simulink model "PMSM_2017b_1013"  (R2017b)
settings: Solver=FixedStepDiscrete  StartTime=0.0  StopTime=0.4  FixedStep=Ts  RelTol=1e-4  EnableMultiTasking=on
values from neighbouring files (symbols this model uses):
  AgSelector = 0    [initialization_1013.m]
  Ba = (Beta*J- Fl)/(1.5*P*flux)    [initialization_1013.m]
  Fl = 0.007*3/(100*pi)    (= 6.68450760986e-05)    [initialization_1013.m]
  flux = Kt/(1.5*P*sqrt(2))    [initialization_1013.m]
  fpwm = 1e4    (= 10000)    [initialization_1013.m]
  Imax = 6*sqrt(2)    [initialization_1013.m]
  J = 9.96e-5    (= 9.96e-05)    [initialization_1013.m]
  K1 = wn^2    (= 1000000)    [initialization_1013.m]
  K2 = 2*fei/wn    (= 0.003)    [initialization_1013.m]
  K_resolver = 1    [initialization_1013.m]
  Ki_Cctrl_d = Rs/(4*Tpwm)    (= 22125)    [initialization_1013.m]
  Ki_Cctrl_q = Rs/(4*Tpwm)    (= 22125)    [initialization_1013.m]
  Ki_Spdctrl = Beta*Kp_Spdctrl    [initialization_1013.m]
  Ki_Spdctrl_2 = 0.12*(pi*J)/(6000*P*flux*Tpwm^2)    [initialization_1013.m]
  Kp_Cctrl_d = Ld/(4*Tpwm)    (= 231.25)    [initialization_1013.m]
  Kp_Cctrl_q = Lq/(4*Tpwm)    (= 231.25)    [initialization_1013.m]
  Kp_Spdctrl = (Beta*J)/(1.5*P*flux)    [initialization_1013.m]
  Kp_Spdctrl_2 = 1*(pi*J)/(300*P*flux*Tpwm)    [initialization_1013.m]
  Kt = 1.32    [initialization_1013.m]
  Ld = Ls    (= 0.0925)    [initialization_1013.m]
  Lq = Ls    (= 0.0925)    [initialization_1013.m]
  Ls = 0.185/2    (= 0.0925)    [initialization_1013.m]
  P = 2    [initialization_1013.m]
  Rs = 17.7/2    (= 8.85)    [initialization_1013.m]
  SimMode = 1    [initialization_1013.m]
  TestCurrentController = 0    [initialization_1013.m]
  Tf = 0.08    [initialization_1013.m]
  Tpwm = 1e-4    (= 0.0001)    [initialization_1013.m]
  TqNorm = 0.6*9550/2500    (= 2.292)    [initialization_1013.m]
  Ts = 1e-6    (= 1e-06)    [initialization_1013.m]
  Udc = 230*sqrt(2)    [initialization_1013.m]
undefined symbols (not defined in the file or in its folder): A, B, DiscIntNeverNeededParam, f_LPF, f_LPF2, Init, K_SMO, Ki, Ki_PLL_SMO, Kp, Kp_PLL_SMO, LowerLimit, rate, UpperLimit
libraries: simulink x11, powerlib x7
(part 2 of 2)

== system PMSM_2017b_1013/SW/AgWeCalculation/Ag_atan2 ==
  Sin : Inport
  cos : Inport  Port=2
  Discrete Derivative : simulink/Discrete/Discrete Derivative  gainval=1.0  ICPrevScaledInput=0.0  OutMin=[]  OutMax=[]  OutDataType=fixdt(1, 16)  OutScaling=2^-10  DoSatur=off
  Sin1 : Trigonometry  Operator=atan2
  Ag : Outport
  we : Outport  Port=2
  wires:
  Sin/1 -> Sin1/1
  Sin1/1 -> Discrete Derivative/1, Ag/1
  Discrete Derivative/1 -> we/1
  cos/1 -> Sin1/2

== system PMSM_2017b_1013/SW/AgWeCalculation/LPF1 ==
  u_in : Inport
  Add : Sum  Inputs=+-
  Add1 : Sum
  Constant : Constant  Value=Tpwm
  Constant1 : Constant  Value=3000/(2*pi)
  Gain3 : Gain  Gain=2*pi
  Product : Product
  Product1 : Product
  Scope_We{1..4} (4 alike) : Scope
  Unit Delay : UnitDelay  SampleTime=-1
  u_out : Outport
  wires:
  Add1/1 -> Unit Delay/1, Scope_We2/1, u_out/1
  Product/1 -> Product1/1
  Add/1 -> Scope_We3/1, Product1/2
  Product1/1 -> Scope_We1/1, Add1/1
  Gain3/1 -> Product/2
  Constant/1 -> Product/1
  Constant1/1 -> Gain3/1
  u_in/1 -> Scope_We4/1, Add/1
  Unit Delay/1 -> Add/2, Add1/2

== system PMSM_2017b_1013/SW/AgWeCalculation/UseRslvrAg ==
  Rslvr_Sin : Inport
  Rslvr_Cos : Inport  Port=2
  Ag_PIcontroller : Subsystem
  Ag_Rslvr : Outport
  We__Rslvr : Outport  Port=2
  wires:
  Rslvr_Sin/1 -> Ag_PIcontroller/1(In1)
  Rslvr_Cos/1 -> Ag_PIcontroller/2(In2)
  Ag_PIcontroller/2(we) -> We__Rslvr/1
  Ag_PIcontroller/1(Ag) -> Ag_Rslvr/1

== system PMSM_2017b_1013/SW/AgWeCalculation/UseSimAg ==
  Agm : Inport
  wm : Inport  Port=2
  Agm2Ag : Gain  Gain=P
  Constant2 : Constant  Value=2*pi
  Mod : Math  Operator=mod  SaturateOnIntegerOverflow=on
  wm2we : Gain  Gain=P
  Ag_sim : Outport
  We_sim : Outport  Port=2
  wires:
  wm2we/1 -> We_sim/1  "we_sim"
  Agm/1 -> Agm2Ag/1
  wm/1 -> wm2we/1
  Agm2Ag/1 -> Mod/1  "Ag_sim"
  Constant2/1 -> Mod/2
  Mod/1 -> Ag_sim/1

== system PMSM_2017b_1013/SW/CurrentController/Anti_Clark ==
  UAlphaBeta : Inport
  Fcn : Fcn  Expr=-0.5*u(1)+sqrt(3)/2*u(2)
  Fcn1 : Fcn  Expr=-0.5*u(1)-sqrt(3)/2*u(2)
  Fcn2 : Fcn  Expr=u(1)
  Mux : Mux  Inputs=3
  Uabc : Outport
  wires:
  UAlphaBeta/1 -> Fcn1/1, Fcn2/1, Fcn/1
  Mux/1 -> Uabc/1
  Fcn2/1 -> Mux/1
  Fcn/1 -> Mux/2
  Fcn1/1 -> Mux/3

== system PMSM_2017b_1013/SW/CurrentController/Anti_Park ==
  Udq : Inport
  Ag : Inport  Port=2
  Constant3 : Constant  Value=1/10000
  ConstantAg : Constant
  Fcn : Fcn  Expr=u(1)*cos(u(3))-u(2)*sin(u(3))
  Fcn1 : Fcn  Expr=u(1)*sin(u(3))+u(2)*cos(u(3))
  Multiport Switch : MultiPortSwitch
  Mux : Mux  Inputs=2
  Mux1 : Mux  Inputs=2
  Mux2 : Mux  Inputs=3
  Sum : Sum  Inputs=|++
  Switch : Switch  Criteria=u2 > Threshold  Threshold=0.5
  SwitchAgForOpenLoop : Constant
  SwitchOpenLoop : Constant  Value=0
  Ud_Inject : Constant  Value=0
  Unit Delay : UnitDelay  SampleTime=-1
  Uq_Inject : Constant  Value=0
  UAlphaBeta : Outport
  wires:
  Udq/1 -> Mux1/1
  Switch/1 -> Fcn1/1, Fcn/1
  Uq_Inject/1 -> Mux2/2
  Mux2/1 -> Switch/1
  Mux1/1 -> Switch/3
  SwitchOpenLoop/1 -> Switch/2
  Ud_Inject/1 -> Mux2/1
  Constant3/1 -> Sum/1
  Unit Delay/1 -> Sum/2
  Sum/1 -> Unit Delay/1, Multiport Switch/3
  Ag/1 -> Multiport Switch/4, Mux1/2
  Fcn/1 -> Mux/1
  Fcn1/1 -> Mux/2
  Mux/1 -> UAlphaBeta/1
  Multiport Switch/1 -> Mux2/3
  SwitchAgForOpenLoop/1 -> Multiport Switch/1
  ConstantAg/1 -> Multiport Switch/2

== system PMSM_2017b_1013/SW/CurrentController/Clamping_PI ==
  Idq_error : Inport
  Udc : Inport  Port=2
  Clamping_PI_d : Subsystem
  Clamping_PI_q : Subsystem
  Constant : Constant  Value=Kp_Cctrl_d
  Constant1 : Constant  Value=Ki_Cctrl_d
  Constant2 : Constant  Value=Kp_Cctrl_q
  Constant3 : Constant  Value=Ki_Cctrl_q
  Demux : Demux  Outputs=2
  Mux : Mux  Inputs=2
  Udq_pi : Outport  InitialOutput=0
  wires:
  Idq_error/1 -> Demux/1
  Demux/1 -> Clamping_PI_d/1(Error)
  Clamping_PI_d/1(Out) -> Mux/1
  Mux/1 -> Udq_pi/1
  Udc/1 -> Clamping_PI_q/2(Udc), Clamping_PI_d/2(Udc)
  Constant/1 -> Clamping_PI_d/3(Kp)
  Constant1/1 -> Clamping_PI_d/4(Ki)
  Clamping_PI_q/1(Out) -> Mux/2
  Constant3/1 -> Clamping_PI_q/4(Ki)
  Constant2/1 -> Clamping_PI_q/3(Kp)
  Demux/2 -> Clamping_PI_q/1(Error)

== system PMSM_2017b_1013/SW/CurrentController/Clark ==
  Iabc : Inport
  Mux1 : Mux  Inputs=2
  alpha : Fcn  Expr=(u(1)-0.5*(u(2)+u(3)))*2/3
  beta : Fcn  Expr=sqrt(3)/2*(u(2)-u(3))*2/3
  I_AlphaBeta : Outport
  wires:
  Iabc/1 -> alpha/1, beta/1
  alpha/1 -> Mux1/1
  beta/1 -> Mux1/2
  Mux1/1 -> I_AlphaBeta/1

== system PMSM_2017b_1013/SW/CurrentController/Decoup ==
  IdqAct : Inport
  we : Inport  Port=2
  Fcn : Fcn  Expr=(u(1)*u(3)*Ld)+(u(3)*flux)
  Fcn1 : Fcn  Expr=-u(2)*u(3)*Lq
  Mux2 : Mux  Inputs=2
  Mux3 : Mux  Inputs=2
  Udq_decp : Outport
  wires:
  we/1 -> Mux2/2
  IdqAct/1 -> Mux2/1
  Fcn1/1 -> Mux3/1
  Fcn/1 -> Mux3/2
  Mux3/1 -> Udq_decp/1
  Mux2/1 -> Fcn1/1, Fcn/1

== system PMSM_2017b_1013/SW/CurrentController/Friction ==
  note: 参考： 摩擦力模型综述 - 豆丁网 (docin.com)
      | 库伦+粘滞摩擦模型： T = Tf * sgn(wm) + Fl*wm
      |
      | 实际转速在0附近会有波动，因此设定一个2rpm的范围，最大静摩擦扭矩与转速成近似线性。
      | 否则实际控制中，0转速会有dq电流在波动。
      |
      | 还有一种解决方案，通过测功机拖动被测电机，测试不同转速下的 摩擦扭矩。最终形成插值表。
      | (该方法对测功机低速控制要求较高)
  we : Inport
  Abs : Abs
  Add : Sum
  Constant : Constant  Value=0
  Divide : Product  Inputs=*/
  Mux1 : Mux  Inputs=2
  Nm->Iq : Gain  Gain=sqrt(2)/Kt
  Product : Product
  Product1 : Product
  Relational Operator : RelationalOperator  OutDataTypeStr=boolean  RndMeth=Simplest
  Rpm2wm : Gain  Gain=pi/30
  RpmThreshold : Constant  Value=2
  Scope1 : Scope
  Scope2 : Scope
  Sign : Signum
  Static : Constant  Value=Tf
  Switch1 : Switch  Criteria=u2 > Threshold  Threshold=0.5
  viscous : Gain  Gain=Fl
  we2wm : Gain  Gain=1/P
  Idq_Friction : Outport
  wires:
  we/1 -> we2wm/1
  viscous/1 -> Add/1
  Mux1/1 -> Idq_Friction/1
  Nm->Iq/1 -> Mux1/2
  Constant/1 -> Mux1/1
  we2wm/1 -> Product1/2, Abs/1, Sign/1, viscous/1, Scope1/1
  Abs/1 -> Relational Operator/1
  Relational Operator/1 -> Switch1/2
  Product/1 -> Add/2
  Add/1 -> Switch1/1
  Switch1/1 -> Scope2/1, Nm->Iq/1
  Sign/1 -> Product/2
  Product1/1 -> Switch1/3
  RpmThreshold/1 -> Divide/2, Rpm2wm/1
  Rpm2wm/1 -> Relational Operator/2
  Static/1 -> Divide/1, Product/1
  Divide/1 -> Product1/1

== system PMSM_2017b_1013/SW/CurrentController/Park ==
  I_AlphaBeta : Inport
  Ag : Inport  Port=2
  Mux : Mux  Inputs=2
  Mux1 : Mux  Inputs=2
  d : Fcn  Expr=u(1)*cos(u(3))+u(2)*sin(u(3))
  q : Fcn  Expr=-u(1)*sin(u(3))+u(2)*cos(u(3))
  IdqAct : Outport
  wires:
  I_AlphaBeta/1 -> Mux/1
  Mux/1 -> q/1, d/1
  Ag/1 -> Mux/2
  d/1 -> Mux1/1
  q/1 -> Mux1/2
  Mux1/1 -> IdqAct/1

== system PMSM_2017b_1013/SW/CurrentController/TqEstimation ==
  IdqAct : Inport
  Demux : Demux  Outputs=2
  Iq2Nm : Gain  Gain=Kt/sqrt(2)
  Scope2 : Scope
  Terminator : Terminator
  TqAct : Outport
  wires:
  Iq2Nm/1 -> TqAct/1, Scope2/1
  IdqAct/1 -> Demux/1
  Demux/2 -> Iq2Nm/1
  Demux/1 -> Terminator/1

== system PMSM_2017b_1013/SW/SVPWM/Sector Caculate ==
  Ualpha : Inport
  Ubeta : Inport  Port=2
  B0 : Fcn  Expr=u[2]
  B1 : Fcn  Expr=u[1]*sqrt(3/4)-0.5*u[2]
  B2 : Fcn  Expr=-u[1]*sqrt(3/4)-u[2]*0.5
  Constant : Constant
  Constant1 : Constant  Value=0
  Mux : Mux  Inputs=2
  Mux1 : Mux  Inputs=3
  N : Fcn  Expr=4*u[3]+2*u[2]+u[1]
  Switch : Switch
  Switch1 : Switch
  Switch2 : Switch
  "N " : Outport
  wires:
  Switch2/1 -> Mux1/3
  Switch/1 -> Mux1/1
  Ualpha/1 -> Mux/1
  Ubeta/1 -> Mux/2
  Mux/1 -> B2/1, B1/1, B0/1
  B0/1 -> Switch/2
  B1/1 -> Switch1/2
  B2/1 -> Switch2/2
  Constant/1 -> Switch/1, Switch2/1, Switch1/1
  Constant1/1 -> Switch/3, Switch1/3, Switch2/3
  Switch1/1 -> Mux1/2
  Mux1/1 -> N/1
  N/1 -> "N "/1

== system PMSM_2017b_1013/SW/SVPWM/T1T1 Caculate ==
  note: T1
  note: T2
  N : Inport
  XYZ : Inport  Port=2
  Tpwm : Inport  Port=3
  Demux : Demux  Outputs=3
  Fcn : Fcn  Expr=u(3)-u(2)-u(1)
  Fcn1 : Fcn  Expr=u(1)*u(3)/(u(1)+u(2))
  Fcn2 : Fcn  Expr=u(2)*u(3)/(u(1)+u(2))
  Gain : Gain  Gain=-1
  Gain1 : Gain  Gain=-1
  Gain2 : Gain  Gain=-1
  Multiport Switch : MultiPortSwitch  Inputs=6  DiagnosticForDefault=Warning
  Multiport Switch1 : MultiPortSwitch  Inputs=6  DiagnosticForDefault=Warning
  Mux : Mux  Inputs=3
  Switch : Switch
  Switch1 : Switch  Criteria=u2 > Threshold
  T1 : Outport
  T2 : Outport  Port=2
  wires:
  Tpwm/1 -> Mux/3
  XYZ/1 -> Demux/1
  Switch1/1 -> T2/1
  Switch/1 -> T1/1
  Fcn2/1 -> Switch1/3
  Fcn1/1 -> Switch/3
  Fcn/1 -> Switch/2, Switch1/2
  Mux/1 -> Fcn1/1, Fcn/1, Fcn2/1
  Multiport Switch/1 -> Switch/1, Mux/1
  Multiport Switch1/1 -> Switch1/1, Mux/2
  N/1 -> Multiport Switch/1, Multiport Switch1/1
  Demux/2 -> Multiport Switch/3, Multiport Switch1/2, Gain1/1
  Demux/3 -> Multiport Switch1/5, Multiport Switch/2, Gain2/1
  Demux/1 -> Multiport Switch/6, Multiport Switch1/4, Gain/1
  Gain/1 -> Multiport Switch1/3, Multiport Switch/5
  Gain2/1 -> Multiport Switch/4, Multiport Switch1/7
  Gain1/1 -> Multiport Switch1/6, Multiport Switch/7

== system PMSM_2017b_1013/SW/SVPWM/Tcm Caculate ==
  N : Inport
  T1 : Inport  Port=2
  T2 : Inport  Port=3
  Tpwm : Inport  Port=4
  Fcn : Fcn  Expr=(u[3]-u[1]-u[2])/4
  Fcn1 : Fcn  Expr=(u[3]+u[1]-u[2])/4
  Fcn2 : Fcn  Expr=(u[3]+u[2]+u[1])/4
  Multiport Switch : MultiPortSwitch  Inputs=6  DiagnosticForDefault=Warning
  Multiport Switch1 : MultiPortSwitch  Inputs=6  DiagnosticForDefault=Warning
  Multiport Switch2 : MultiPortSwitch  Inputs=6  DiagnosticForDefault=Warning
  Mux : Mux  Inputs=3
  Mux1 : Mux  Inputs=3
  Tcm1 Tcm2 Tcm3 : Outport
  wires:
  Mux/1 -> Fcn2/1, Fcn/1, Fcn1/1
  Tpwm/1 -> Mux/3
  T2/1 -> Mux/2
  T1/1 -> Mux/1
  Multiport Switch2/1 -> Mux1/3
  Multiport Switch1/1 -> Mux1/2
  Multiport Switch/1 -> Mux1/1
  Mux1/1 -> Tcm1 Tcm2 Tcm3/1
  Fcn/1 -> Multiport Switch/3, Multiport Switch/4, Multiport Switch1/6, Multiport Switch2/5, Multiport Switch2/7, Multiport Switch1/2
  Fcn1/1 -> Multiport Switch1/5, Multiport Switch2/3, Multiport Switch2/6, Multiport Switch1/4, Multiport Switch/7, Multiport Switch/2
  Fcn2/1 -> Multiport Switch/5, Multiport Switch/6, Multiport Switch1/3, Multiport Switch1/7, Multiport Switch2/2, Multiport Switch2/4
  N/1 -> Multiport Switch2/1, Multiport Switch1/1, Multiport Switch/1

== system PMSM_2017b_1013/SW/SVPWM/XYZ Caculate ==
  Ualpha : Inport
  Ubeta : Inport  Port=2
  Tpwm : Inport  Port=3
  Udc : Inport  Port=4
  Add : Sum
  Add1 : Sum  Inputs=+-
  Gain : Gain  Gain=3/2
  Gain1 : Gain  Gain=sqrt(3)
  Gain2 : Gain  Gain=sqrt(3)/2
  Math Function : Math  Operator=reciprocal  SaturateOnIntegerOverflow=on
  Mux : Mux  Inputs=3
  Product{,1..3} (4 alike) : Product  RndMeth=Zero
  XYZ : Outport
  wires:
  Mux/1 -> XYZ/1
  Product1/1 -> Mux/1
  Product3/1 -> Mux/2
  Product2/1 -> Mux/3
  Ualpha/1 -> Gain/1
  Ubeta/1 -> Gain2/1, Gain1/1
  Udc/1 -> Math Function/1
  Math Function/1 -> Product/2
  Tpwm/1 -> Product/1
  Gain1/1 -> Product1/1
  Product/1 -> Product2/2, Product1/2, Product3/2
  Gain/1 -> Add1/2, Add/2
  Gain2/1 -> Add/1, Add1/1
  Add1/1 -> Product2/1
  Add/1 -> Product3/1

== system PMSM_2017b_1013/SW/SpdController/Clamping_PI ==
  Spd_error : Inport
  SpdAct : Inport  Port=2
  Clamping_PI_Spd : Subsystem
  Constant : Constant  Value=Kp_Spdctrl
  Constant1 : Constant  Value=Ki_Spdctrl
  Constant2 : Constant  Value=Imax
  Gain : Gain  Gain=Ba
  Gain1 : Gain  Gain=pi/30
  Gain2 : Gain  Gain=pi/30
  IqReq : Outport  InitialOutput=0
  wires:
  Clamping_PI_Spd/1(Out) -> IqReq/1
  Constant/1 -> Clamping_PI_Spd/3(Kp)
  Constant1/1 -> Clamping_PI_Spd/4(Ki)
  Constant2/1 -> Clamping_PI_Spd/2(Imax)
  SpdAct/1 -> Gain1/1
  Gain/1 -> Clamping_PI_Spd/5(SpdAct)
  Spd_error/1 -> Gain2/1
  Gain1/1 -> Gain/1
  Gain2/1 -> Clamping_PI_Spd/1(Error)

== system PMSM_2017b_1013/SW/SpdController/Clamping_PI1 ==
  Spd_error : Inport
  Clamping_PI_Spd : Subsystem
  Constant : Constant  Value=Kp_Spdctrl_2
  Constant1 : Constant  Value=Ki_Spdctrl_2
  Constant2 : Constant  Value=Imax
  Nr2wm : Gain  Gain=pi/30
  IqReq : Outport  InitialOutput=0
  wires:
  Nr2wm/1 -> Clamping_PI_Spd/1(Error)
  Constant2/1 -> Clamping_PI_Spd/2(Imax)
  Spd_error/1 -> Nr2wm/1
  Constant1/1 -> Clamping_PI_Spd/4(Ki)
  Constant/1 -> Clamping_PI_Spd/3(Kp)
  Clamping_PI_Spd/1(Out) -> IqReq/1

== system PMSM_2017b_1013/SW/SpdController/EOT ==
  note: 采用Id=0控制
  IqReq : Inport
  IdReq : Constant  Value=0
  Mux : Mux  Inputs=2
  IdqReq : Outport
  wires:
  IqReq/1 -> Mux/2
  IdReq/1 -> Mux/1
  Mux/1 -> IdqReq/1

== system PMSM_2017b_1013/Development Lib/UseMRASAg/MRAS/Subsystem ==
  ud : Inport
  uq : Inport  Port=2
  we : Inport  Port=3
  1/L : Gain  Gain=1/0.000395
  1/L1 : Gain  Gain=1/0.000395
  F/L : Gain  Gain=0.1194/0.000395
  Integrator : Integrator
  Integrator1 : Integrator
  Product : Product  RndMeth=Zero
  Product1 : Product  RndMeth=Zero
  R/L : Gain  Gain=0.0485/0.000395
  R/L1 : Gain  Gain=0.0485/0.000395
  Subtract : Sum  Inputs=---+
  Subtract1 : Sum  Inputs=+-+
  i_d : Outport
  i_q : Outport  Port=2
  wires:
  1/L1/1 -> Subtract/4
  we/1 -> F/L/1, Product/2, Product1/1
  R/L/1 -> Subtract1/2
  Product/1 -> Subtract/1
  R/L1/1 -> Subtract/3
  Subtract1/1 -> Integrator1/1
  Subtract/1 -> Integrator/1
  1/L/1 -> Subtract1/1
  Product1/1 -> Subtract1/3
  F/L/1 -> Subtract/2
  ud/1 -> 1/L/1
  uq/1 -> 1/L1/1
  Integrator1/1 -> Product/1, i_d/1, R/L/1
  Integrator/1 -> R/L1/1, Product1/2, i_q/1

== system PMSM_2017b_1013/Development Lib/UseMRASAg/MRAS/Subsystem1 ==
  id : Inport
  iq : Inport  Port=2
  i_d1 : Inport  Port=3
  i_q1 : Inport  Port=4
  F/L : Gain  Gain=0.1194/0.000395
  Integrator : Integrator
  Ki : Gain  Gain=0.001
  Kp : Gain  Gain=0.1
  Memory : Memory
  Product2 : Product  RndMeth=Zero
  Product3 : Product  RndMeth=Zero
  Subtract1 : Sum  Inputs=+--
  Subtract2 : Sum
  Subtract3 : Sum  Inputs=+-
  w_e : Outport
  wires:
  id/1 -> Product2/1
  i_q1/1 -> Product2/2, Subtract3/2
  Subtract1/1 -> Ki/1, Kp/1
  i_d1/1 -> Product3/2
  Ki/1 -> Integrator/1
  Product2/1 -> Subtract1/1
  F/L/1 -> Subtract1/3
  Integrator/1 -> Subtract2/1
  Product3/1 -> Subtract1/2
  iq/1 -> Product3/1, Subtract3/1
  Subtract3/1 -> F/L/1
  Kp/1 -> Subtract2/2
  Subtract2/1 -> Memory/1
  Memory/1 -> w_e/1

== system PMSM_2017b_1013/Development Lib/UseMRASAg/MRAS/change theta ==
  In1 : Inport
  Constant : Constant  Value=2*pi
  Constant2 : Constant  Value=0
  Math Function : Math  Operator=mod  SaturateOnIntegerOverflow=on
  Step2 : Step  Time=0.002  After=2  SampleTime=0
  Switch : Switch  Criteria=u2 > Threshold  Threshold=1
  Out1 : Outport
  wires:
  Constant/1 -> Math Function/2
  Constant2/1 -> Switch/3
  Step2/1 -> Switch/2
  In1/1 -> Math Function/1
  Math Function/1 -> Switch/1
  Switch/1 -> Out1/1

== system PMSM_2017b_1013/Development Lib/UseSMOAg/PLL /LPF ==
  u_in : Inport
  Add : Sum  Inputs=+-
  Add1 : Sum
  Constant : Constant  Value=Tpwm
  Constant1 : Constant  Value=f_LPF
  Gain3 : Gain  Gain=2*pi
  Product : Product
  Product1 : Product
  Unit Delay : UnitDelay  SampleTime=-1
  u_out : Outport
  wires:
  Unit Delay/1 -> Add1/2, Add/2
  u_in/1 -> Add/1
  Constant1/1 -> Gain3/1
  Constant/1 -> Product/1
  Gain3/1 -> Product/2
  Product1/1 -> Add1/1
  Add/1 -> Product1/2
  Product/1 -> Product1/1
  Add1/1 -> u_out/1, Unit Delay/1

== system PMSM_2017b_1013/Development Lib/UseSMOAg/PLL /Subsystem ==
  e : Inport
  Add1 : Sum
  Discrete-Time Integrator1 : DiscreteIntegrator  SampleTime=-1  ICPrevOutput=DiscIntNeverNeededParam  ICPrevScaledInput=DiscIntNeverNeededParam
  Gain1 : Gain  Gain=Kp_PLL_SMO
  Gain2 : Gain  Gain=Ki_PLL_SMO
  Zero-Order Hold1 : ZeroOrderHold  SampleTime=-1
  Out1 : Outport
  wires:
  Gain2/1 -> Discrete-Time Integrator1/1
  Gain1/1 -> Zero-Order Hold1/1
  e/1 -> Gain2/1, Gain1/1
  Discrete-Time Integrator1/1 -> Add1/2
  Add1/1 -> Out1/1
  Zero-Order Hold1/1 -> Add1/1

== system PMSM_2017b_1013/Development Lib/UseSMOAg/Subsystem/Clark1 ==
  Iabc : Inport
  Mux1 : Mux  Inputs=2
  alpha : Fcn  Expr=(u(1)-0.5*(u(2)+u(3)))*2/3
  beta : Fcn  Expr=sqrt(3)/2*(u(2)-u(3))*2/3
  I_AlphaBeta : Outport
  wires:
  Iabc/1 -> alpha/1, beta/1
  alpha/1 -> Mux1/1
  beta/1 -> Mux1/2
  Mux1/1 -> I_AlphaBeta/1

== system PMSM_2017b_1013/Development Lib/UseSMOAg/Subsystem/Clark2 ==
  Iabc : Inport
  Mux1 : Mux  Inputs=2
  alpha : Fcn  Expr=(u(1)-0.5*(u(2)+u(3)))*2/3
  beta : Fcn  Expr=sqrt(3)/2*(u(2)-u(3))*2/3
  I_AlphaBeta : Outport
  wires:
  Mux1/1 -> I_AlphaBeta/1
  beta/1 -> Mux1/2
  alpha/1 -> Mux1/1
  Iabc/1 -> beta/1, alpha/1

== system PMSM_2017b_1013/Development Lib/UseSMOAg/Subsystem/LPF ==
  u_in : Inport
  Add : Sum  Inputs=+-
  Add1 : Sum
  Constant : Constant  Value=Tpwm
  Constant1 : Constant  Value=f_LPF
  Gain3 : Gain  Gain=2*pi
  Product : Product
  Product1 : Product
  Unit Delay : UnitDelay  SampleTime=-1
  u_out : Outport
  wires:
  Unit Delay/1 -> Add1/2, Add/2
  u_in/1 -> Add/1
  Constant1/1 -> Gain3/1
  Constant/1 -> Product/1
  Gain3/1 -> Product/2
  Product1/1 -> Add1/1
  Add/1 -> Product1/2
  Product/1 -> Product1/1
  Add1/1 -> u_out/1, Unit Delay/1

== system PMSM_2017b_1013/Development Lib/UseSMOAg/Subsystem/LPF1 ==
  u_in : Inport
  Add : Sum  Inputs=+-
  Add1 : Sum
  Constant : Constant  Value=Tpwm
  Constant1 : Constant  Value=f_LPF
  Gain3 : Gain  Gain=2*pi
  Product : Product
  Product1 : Product
  Unit Delay : UnitDelay  SampleTime=-1
  u_out : Outport
  wires:
  Add1/1 -> Unit Delay/1, u_out/1
  Product/1 -> Product1/1
  Add/1 -> Product1/2
  Product1/1 -> Add1/1
  Gain3/1 -> Product/2
  Constant/1 -> Product/1
  Constant1/1 -> Gain3/1
  u_in/1 -> Add/1
  Unit Delay/1 -> Add/2, Add1/2

== system PMSM_2017b_1013/Offline Parameter Identification/RLS/RLS/Ls ==
  phi : Inport
  Rou : Inport  Port=2
  Add : Sum  Inputs=+-
  Divide5 : Product  Inputs=*/  Multiplication=Matrix(*)
  Product of Elements2 : Product  Inputs=3  Multiplication=Matrix(*)
  Product of Elements4 : Product  Inputs=3  Multiplication=Matrix(*)
  Product of Elements5 : Product  Multiplication=Matrix(*)
  Product of Elements7 : Product  Inputs=*/
  Reshape : Reshape  OutputDimensionality=Customize
  Sum2 : Sum  Inputs=|++
  Unit Delay : UnitDelay  InitialCondition=100  SampleTime=-1
  G : Outport
  wires:
  Reshape/1 -> Product of Elements4/1, Product of Elements2/2  "phiT"
  phi/1 -> Reshape/1, Product of Elements5/2, Product of Elements4/3
  Rou/1 -> Product of Elements7/2, Sum2/2
  Add/1 -> Product of Elements7/1
  Product of Elements7/1 -> Unit Delay/1  "p"
  Divide5/1 -> G/1, Product of Elements2/1  "G"
  Sum2/1 -> Divide5/2
  Unit Delay/1 -> Add/1, Product of Elements4/2, Product of Elements5/1, Product of Elements2/3
  Product of Elements5/1 -> Divide5/1
  Product of Elements4/1 -> Sum2/1
  Product of Elements2/1 -> Add/2

== system PMSM_2017b_1013/Offline Parameter Identification/RLS/RLS/Rs_flux ==
  phi : Inport
  Rou : Inport  Port=2
  Add : Sum  Inputs=+-
  Divide5 : Product  Inputs=*/  Multiplication=Matrix(*)
  Product of Elements2 : Product  Inputs=3  Multiplication=Matrix(*)
  Product of Elements4 : Product  Inputs=3  Multiplication=Matrix(*)
  Product of Elements5 : Product  Multiplication=Matrix(*)
  Product of Elements7 : Product  Inputs=*/
  Reshape : Reshape  OutputDimensionality=Customize  OutputDimensions=[1,2]
  Sum2 : Sum  Inputs=|++
  Unit Delay : UnitDelay  InitialCondition=0.0009*eye(2)  SampleTime=-1
  G : Outport
  wires:
  Reshape/1 -> Product of Elements4/1, Product of Elements2/2  "phiT"
  phi/1 -> Reshape/1, Product of Elements5/2, Product of Elements4/3
  Rou/1 -> Product of Elements7/2, Sum2/2
  Add/1 -> Product of Elements7/1
  Product of Elements7/1 -> Unit Delay/1  "p"
  Divide5/1 -> G/1, Product of Elements2/1  "G"
  Sum2/1 -> Divide5/2
  Unit Delay/1 -> Add/1, Product of Elements4/2, Product of Elements5/1, Product of Elements2/3
  Product of Elements5/1 -> Divide5/1
  Product of Elements4/1 -> Sum2/1
  Product of Elements2/1 -> Add/2

== system PMSM_2017b_1013/SW/AgWeCalculation/UseRslvrAg/Ag_PIcontroller ==
  In1 : Inport
  In2 : Inport  Port=2
  Add : Sum  Inputs=+-
  Add1 : Sum
  Constant2 : Constant  Value=2*pi
  Discrete-Time Integrator : DiscreteIntegrator  IntegratorMethod=Integration: Backward Euler  SampleTime=-1  ICPrevOutput=DiscIntNeverNeededParam  ICPrevScaledInput=DiscIntNeverNeededParam
  Discrete-Time Integrator1 : DiscreteIntegrator  IntegratorMethod=Integration: Backward Euler  SampleTime=-1  ICPrevOutput=DiscIntNeverNeededParam  ICPrevScaledInput=DiscIntNeverNeededParam
  Gain : Gain  Gain=K1
  Gain1 : Gain  Gain=K2
  Mod : Math  Operator=mod  SaturateOnIntegerOverflow=on
  Product : Product
  Product1 : Product
  Sin : Trigonometry
  Sin1 : Trigonometry  Operator=cos
  Ag : Outport
  we : Outport  Port=2
  wires:
  In2/1 -> Product1/1
  Gain/1 -> Discrete-Time Integrator/1
  Discrete-Time Integrator/1 -> we/1, Gain1/1, Discrete-Time Integrator1/1
  Gain1/1 -> Add1/2
  Discrete-Time Integrator1/1 -> Add1/1
  Product1/1 -> Add/2
  Sin1/1 -> Product/2
  Sin/1 -> Product1/2
  Add/1 -> Gain/1  "e"
  Product/1 -> Add/1
  In1/1 -> Product/1
  Add1/1 -> Mod/1, Sin1/1, Sin/1
  Constant2/1 -> Mod/2
  Mod/1 -> Ag/1

== system PMSM_2017b_1013/SW/CurrentController/Clamping_PI/Clamping_PI_d ==
  Error : Inport
  Udc : Inport  Port=2
  Kp : Inport  Port=3
  Ki : Inport  Port=4
  Abs : Abs
  Constant : Constant
  Constant1 : Constant  Value=0
  Discrete-Time Integrator : DiscreteIntegrator  SampleTime=-1  UpperSaturationLimit=UpperLimit  LowerSaturationLimit=LowerLimit  ICPrevOutput=DiscIntNeverNeededParam  ICPrevScaledInput=DiscIntNeverNeededParam
  Gain : Gain  Gain=1/sqrt(3)
  Gain1 : Gain  Gain=-1
  Product : Product
  Product1 : Product
  Product2 : Product
  Relational Operator : RelationalOperator  Operator=<=  OutDataTypeStr=boolean  RndMeth=Simplest
  Saturation Dynamic : simulink/Discontinuities/Saturation Dynamic  OutMin=[]  OutMax=[]  OutDataTypeStr=Inherit: Same as second input  OutDataType=fixdt(1, 16)  OutScaling=2^-10  DoSatur=off
  Scope2 : Scope
  Sum6 : Sum  InputSameDT=on  OutDataTypeStr=Inherit: Same as first input
  Switch : Switch  Criteria=u2 > Threshold  Threshold=0.5
  Zero-Order Hold : ZeroOrderHold  SampleTime=-1
  Out : Outport  InitialOutput=0
  wires:
  Zero-Order Hold/1 -> Sum6/1
  Product1/1 -> Zero-Order Hold/1
  Sum6/1 -> Saturation Dynamic/2, Abs/1
  Discrete-Time Integrator/1 -> Sum6/2
  Udc/1 -> Gain/1
  Gain/1 -> Saturation Dynamic/1, Relational Operator/2, Gain1/1
  Saturation Dynamic/1 -> Out/1
  Relational Operator/1 -> Switch/2
  Constant1/1 -> Switch/3
  Constant/1 -> Switch/1
  Switch/1 -> Scope2/1, Product/2
  Error/1 -> Product2/1, Product1/2
  Product/1 -> Discrete-Time Integrator/1
  Gain1/1 -> Saturation Dynamic/3
  Product2/1 -> Product/1
  Kp/1 -> Product1/1
  Ki/1 -> Product2/2
  Abs/1 -> Relational Operator/1

== system PMSM_2017b_1013/SW/CurrentController/Clamping_PI/Clamping_PI_q ==
  Error : Inport
  Udc : Inport  Port=2
  Kp : Inport  Port=3
  Ki : Inport  Port=4
  Abs : Abs
  Constant : Constant
  Constant1 : Constant  Value=0
  Discrete-Time Integrator : DiscreteIntegrator  SampleTime=-1  UpperSaturationLimit=UpperLimit  LowerSaturationLimit=LowerLimit  ICPrevOutput=DiscIntNeverNeededParam  ICPrevScaledInput=DiscIntNeverNeededParam
  Gain : Gain  Gain=1/sqrt(3)
  Gain1 : Gain  Gain=-1
  Product : Product
  Product1 : Product
  Product2 : Product
  Relational Operator : RelationalOperator  Operator=<=  OutDataTypeStr=boolean  RndMeth=Simplest
  Saturation Dynamic : simulink/Discontinuities/Saturation Dynamic  OutMin=[]  OutMax=[]  OutDataTypeStr=Inherit: Same as second input  OutDataType=fixdt(1, 16)  OutScaling=2^-10  DoSatur=off
  Scope2 : Scope
  Sum6 : Sum  InputSameDT=on  OutDataTypeStr=Inherit: Same as first input
  Switch : Switch  Criteria=u2 > Threshold  Threshold=0.5
  Zero-Order Hold : ZeroOrderHold  SampleTime=-1
  Out : Outport  InitialOutput=0
  wires:
  Abs/1 -> Relational Operator/1
  Ki/1 -> Product2/2
  Kp/1 -> Product1/1
  Product2/1 -> Product/1
  Gain1/1 -> Saturation Dynamic/3
  Product/1 -> Discrete-Time Integrator/1
  Error/1 -> Product1/2, Product2/1
  Switch/1 -> Product/2, Scope2/1
  Constant/1 -> Switch/1
  Constant1/1 -> Switch/3
  Relational Operator/1 -> Switch/2
  Saturation Dynamic/1 -> Out/1
  Gain/1 -> Gain1/1, Relational Operator/2, Saturation Dynamic/1
  Udc/1 -> Gain/1
  Discrete-Time Integrator/1 -> Sum6/2
  Sum6/1 -> Abs/1, Saturation Dynamic/2
  Product1/1 -> Zero-Order Hold/1
  Zero-Order Hold/1 -> Sum6/1

== system PMSM_2017b_1013/SW/SpdController/Clamping_PI/Clamping_PI_Spd ==
  Error : Inport
  Imax : Inport  Port=2
  Kp : Inport  Port=3
  Ki : Inport  Port=4
  SpdAct : Inport  Port=5
  Abs : Abs
  Constant : Constant
  Constant1 : Constant  Value=0
  Discrete-Time Integrator : DiscreteIntegrator  SampleTime=-1  UpperSaturationLimit=UpperLimit  LowerSaturationLimit=LowerLimit  ICPrevOutput=DiscIntNeverNeededParam  ICPrevScaledInput=DiscIntNeverNeededParam
  Gain1 : Gain  Gain=-1
  Product : Product
  Product1 : Product
  Product2 : Product
  Relational Operator : RelationalOperator  Operator=<=  OutDataTypeStr=boolean  RndMeth=Simplest
  Saturation Dynamic : simulink/Discontinuities/Saturation Dynamic  OutMin=[]  OutMax=[]  OutDataTypeStr=Inherit: Same as second input  OutDataType=fixdt(1, 16)  OutScaling=2^-10  DoSatur=off
  Scope2 : Scope
  Sum6 : Sum  Inputs=++-  InputSameDT=on  OutDataTypeStr=Inherit: Same as first input
  Switch : Switch  Criteria=u2 > Threshold  Threshold=0.5
  Unit Delay : UnitDelay  SampleTime=-1
  Zero-Order Hold : ZeroOrderHold  SampleTime=-1
  Out : Outport  InitialOutput=0
  wires:
  Zero-Order Hold/1 -> Sum6/1
  Product1/1 -> Zero-Order Hold/1
  Sum6/1 -> Saturation Dynamic/2, Abs/1
  Discrete-Time Integrator/1 -> Sum6/2
  Imax/1 -> Saturation Dynamic/1, Relational Operator/2, Gain1/1
  Saturation Dynamic/1 -> Out/1
  Relational Operator/1 -> Switch/2
  Constant1/1 -> Switch/3
  Constant/1 -> Switch/1
  Switch/1 -> Scope2/1, Unit Delay/1
  Error/1 -> Product2/1, Product1/2
  Product/1 -> Discrete-Time Integrator/1
  Gain1/1 -> Saturation Dynamic/3
  Product2/1 -> Product/1
  Kp/1 -> Product1/1
  Ki/1 -> Product2/2
  Abs/1 -> Relational Operator/1
  Unit Delay/1 -> Product/2
  SpdAct/1 -> Sum6/3

== system PMSM_2017b_1013/SW/SpdController/Clamping_PI1/Clamping_PI_Spd ==
  Error : Inport
  Imax : Inport  Port=2
  Kp : Inport  Port=3
  Ki : Inport  Port=4
  Abs : Abs
  Constant : Constant
  Constant1 : Constant  Value=0
  Discrete-Time Integrator : DiscreteIntegrator  IntegratorMethod=Integration: Trapezoidal  SampleTime=-1  UpperSaturationLimit=UpperLimit  LowerSaturationLimit=LowerLimit  ICPrevOutput=DiscIntNeverNeededParam  ICPrevScaledInput=DiscIntNeverNeededParam
  Gain1 : Gain  Gain=-1
  Product : Product
  Product1 : Product
  Product2 : Product
  Relational Operator : RelationalOperator  Operator=<=  OutDataTypeStr=boolean  RndMeth=Simplest
  Saturation Dynamic : simulink/Discontinuities/Saturation Dynamic  OutMin=[]  OutMax=[]  OutDataTypeStr=Inherit: Same as second input  OutDataType=fixdt(1, 16)  OutScaling=2^-10  DoSatur=off
  Scope2 : Scope
  Sum6 : Sum  InputSameDT=on  OutDataTypeStr=Inherit: Same as first input
  Switch : Switch  Criteria=u2 > Threshold  Threshold=0.5
  Unit Delay : UnitDelay  SampleTime=-1
  Zero-Order Hold : ZeroOrderHold  SampleTime=-1
  Out : Outport  InitialOutput=0
  wires:
  Unit Delay/1 -> Product/2
  Abs/1 -> Relational Operator/1
  Ki/1 -> Product2/2
  Kp/1 -> Product1/1
  Product2/1 -> Product/1
  Gain1/1 -> Saturation Dynamic/3
  Product/1 -> Discrete-Time Integrator/1
  Error/1 -> Product1/2, Product2/1
  Switch/1 -> Unit Delay/1, Scope2/1
  Constant/1 -> Switch/1
  Constant1/1 -> Switch/3
  Relational Operator/1 -> Switch/2
  Saturation Dynamic/1 -> Out/1
  Imax/1 -> Gain1/1, Relational Operator/2, Saturation Dynamic/1
  Discrete-Time Integrator/1 -> Sum6/2
  Sum6/1 -> Abs/1, Saturation Dynamic/2
  Product1/1 -> Zero-Order Hold/1
  Zero-Order Hold/1 -> Sum6/1
